simulink model "dom_sim"  (R2014a)
settings: Solver=ode45  StartTime=0.0  StopTime=27000000  RelTol=1e-3
values from neighbouring files (symbols this model uses):
  Cpw = 4190    [blok.m]    (also in dom.m)
  Cvg = Cpw*Rw*Vw    (= 838000)    [blok.m]    (also in dom.m = 628500000)
  Cvk = Cpp*Rw*Vk    (= 201000)    [blok.m]    (also in dom.m = 2010000)
  Cvw = (Cvw1+Cvs)/2    [blok.m]    (also in dom.m = 2347.68)
  dfg = 0    [dom.m]
  dTgz = 0    [dom.m]
  dTzew = 0    [blok.m]    (also in dom.m)
  fg0 = fgN    (= 0.000119331742243)    [dom.m]
  fk0 = fkN    (= 0.000119331742243)    [dom.m]
  Kcg = PgN/(TgpN-TwewN)    (= 200)    [dom.m]
  Kcw = PgN/(TwewN-TzewN)    (= 250)    [dom.m]
  qk0 = x(6,1)    [blok.m]    (also in dom.m = 10000)
  Rw = 1000    [blok.m]    (also in dom.m)
  Tgp0 = Kcw*(Twew0-Tzew0)/Kcg+Twew0    (= 70)    [dom.m]
  Tgz0 = TgzN    (= 90)    [dom.m]
  Tkp0 = TkpN    (= 70)    [dom.m]
  Tkz0 = x(5,1)    [blok.m]    (also in dom.m = 90)
  Twew0 = (Cpw*fmg*Kcg*Tgz0+Kcw*(Kcg+Cpw*fmg)*Tzew0)/(Kcg*Kcw+Cpw*fmg*(Kcg+Kcw))    (= 20)    [dom.m]
  Tzew0 = TzewN    (= -20)    [blok.m]    (also in dom.m)
settings Model: Creator=LAB320-1552  LastModifiedBy=Adrian
settings DebuggingCC: UnderspecifiedInitializationDetection=Classic  SolverPrmCheckMsg=none  StateNameClashWarn=warning

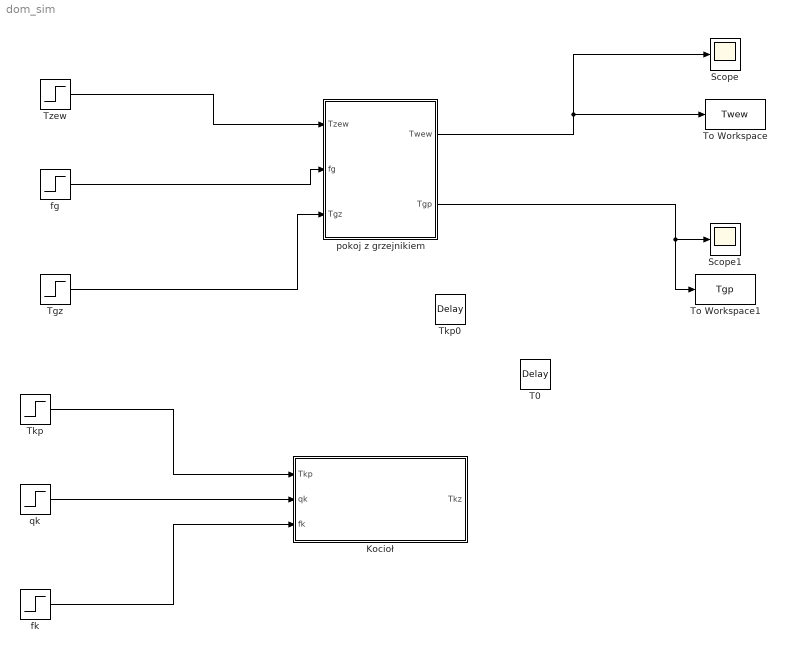
== system dom_sim ==
  Kocioł : Subsystem  mask{Cpw=Cpw, Rw=Rw, Cvk=Cvk, Tz0=Tkz0}
      mask prompts: Tz0 "Tkz0"
  Scope : Scope
      settings: YMin=26.335  YMax=26.3625
  Scope1 : Scope
  T0 : TransportDelay  InitialOutput=Tkz0
  "Tgz " : Step  Before=Tgz0  After=Tgz0+dTgz  SampleTime=0
  Tkp : Step  Before=Tkp0  After=Tkp0  SampleTime=0
  Tkp0 : TransportDelay  InitialOutput=Tkp0
  To Workspace : ToWorkspace  VariableName=Twew  SaveFormat=Timeseries  SampleTime=-1
  To Workspace1 : ToWorkspace  VariableName=Tgp  SaveFormat=Timeseries  SampleTime=-1
  "Tzew " : Step  Before=Tzew0  After=Tzew0+dTzew  SampleTime=0
  "fg " : Step  Before=fg0  After=fg0+dfg  SampleTime=0
  fk : Step  Before=fk0  After=fk0  SampleTime=0
  "pokoj z grzejnikiem " : Subsystem  mask{Kcg=Kcg, Kcw=Kcw, Cvw=Cvw, Cvg=Cvg, Twew0=Twew0, Tgp0=Tgp0, Cpw=Cpw, Rw=Rw}
  qk : Step  Before=qk0  After=qk0  SampleTime=0
  wires:
  "pokoj z grzejnikiem "/2(Tgp) -> To Workspace1/1, Scope1/1
  "pokoj z grzejnikiem "/1(Twew) -> Scope/1, To Workspace/1
  "Tzew "/1 -> "pokoj z grzejnikiem "/1(Tzew)
  "fg "/1 -> "pokoj z grzejnikiem "/2(fg)
  "Tgz "/1 -> "pokoj z grzejnikiem "/3(Tgz)
  Tkp/1 -> Kocioł/1(Tkp)
  qk/1 -> Kocioł/2(qk)
  fk/1 -> Kocioł/3(fk)

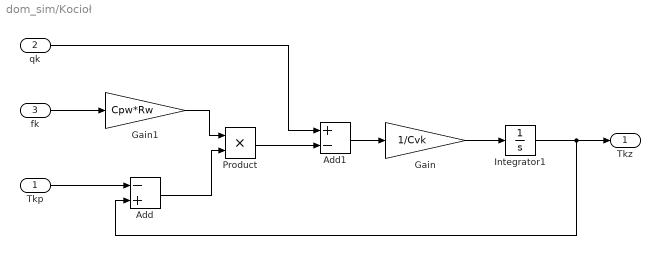
== system dom_sim/Kocioł ==
  Tkp : Inport
  qk : Inport  Port=2
  fk : Inport  Port=3
  Add : Sum  Inputs=-+
  Add1 : Sum  Inputs=+-
  Gain : Gain  Gain=1/Cvk
  Gain1 : Gain  Gain=Cpw*Rw
  Integrator1 : Integrator  InitialCondition=Tkz0
  Product : Product
  Tkz : Outport
  wires:
  Gain/1 -> Integrator1/1
  Integrator1/1 -> Add/2, Tkz/1
  Tkp/1 -> Add/1
  fk/1 -> Gain1/1
  Gain1/1 -> Product/1
  Add/1 -> Product/2
  qk/1 -> Add1/1
  Product/1 -> Add1/2
  Add1/1 -> Gain/1

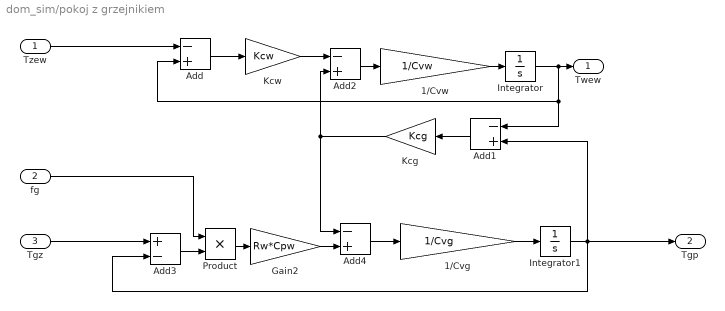
== system dom_sim/pokoj z grzejnikiem  ==
  Tzew : Inport
  fg : Inport  Port=2
  Tgz : Inport  Port=3
  1/Cvg : Gain  Gain=1/Cvg
  1/Cvw : Gain  Gain=1/Cvw
  Add{,1..2,4} (4 alike) : Sum  Inputs=-+
  Add3 : Sum  Inputs=+-
  Gain2 : Gain  Gain=Rw*Cpw
  Integrator : Integrator  InitialCondition=Twew0
  Integrator1 : Integrator  InitialCondition=Tgp0
  "Kcg " : Gain  Gain=Kcg
  Kcw : Gain  Gain=Kcw
  Product : Product
  Twew : Outport
  Tgp : Outport  Port=2
  wires:
  fg/1 -> Product/1
  Kcw/1 -> Add2/1
  1/Cvg/1 -> Integrator1/1
  "Kcg "/1 -> Add4/1, Add2/2
  Add/1 -> Kcw/1
  Add2/1 -> 1/Cvw/1
  1/Cvw/1 -> Integrator/1
  Tzew/1 -> Add/1
  Add4/1 -> 1/Cvg/1
  Gain2/1 -> Add4/2
  Add3/1 -> Product/2
  Tgz/1 -> Add3/1
  Product/1 -> Gain2/1
  Add1/1 -> "Kcg "/1
  Integrator1/1 -> Tgp/1, Add1/2, Add3/2
  Integrator/1 -> Add1/1, Add/2, Twew/1
